simulink model "signal_processing"  (R2026a)
settings: Solver=ode4  StopTime=2.0  FixedStep=0.001
undefined symbols (not defined in the file): LPF_den, LPF_num, Sensor_Noise_Std, Ts
settings Model: Creator=anh  LastModifiedBy=anh
settings DataIOCC: ExternalInput=v_wheel_true_input, v_veh_zero  LoadExternalInput=on

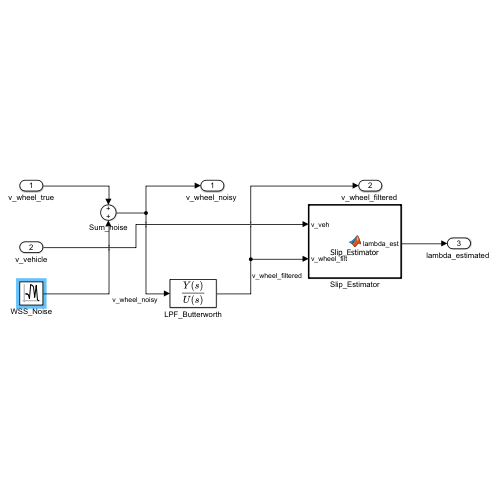
[thumbnail: Simulink's stored preview of the top-level diagram]
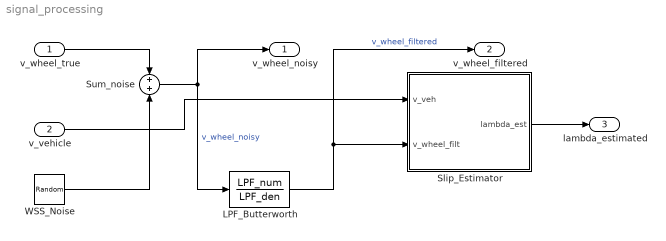
== system signal_processing ==
  v_wheel_true : Inport
  v_vehicle : Inport  Port=2
  LPF_Butterworth : TransferFcn  Numerator=LPF_num  Denominator=LPF_den
  Slip_Estimator : MATLAB Function  TreatAsAtomicUnit=on
  Sum_noise : Sum
  WSS_Noise : RandomNumber  Variance=Sensor_Noise_Std^2  SampleTime=Ts
  "v_wheel_noisy " : Outport
  "v_wheel_filtered " : Outport  Port=2
  "lambda_estimated " : Outport  Port=3
  wires:
  v_wheel_true/1 -> Sum_noise/1
  WSS_Noise/1 -> Sum_noise/2
  Sum_noise/1 -> LPF_Butterworth/1, "v_wheel_noisy "/1  "v_wheel_noisy"
  v_vehicle/1 -> Slip_Estimator/1(v_veh)
  LPF_Butterworth/1 -> "v_wheel_filtered "/1, Slip_Estimator/2(v_wheel_filt)  "v_wheel_filtered"
  Slip_Estimator/1(lambda_est) -> "lambda_estimated "/1

== matlab function signal_processing/Slip_Estimator ==
  data: v_veh input; lambda_est output; v_wheel_filt input
function lambda_est = Slip_Estimator(v_veh, v_wheel_filt)
% SLIP_ESTIMATOR Ước lượng slip ratio từ tín hiệu đã lọc nhiễu
% Có bảo vệ chống chia cho 0 khi xe dừng hẳn

if v_veh < 0.1
    lambda_est = 0.0;
else
    lambda_est = (v_veh - v_wheel_filt) / v_veh;
end

% Clamp về khoảng vật lý [0, 1]
lambda_est = max(0.0, min(1.0, lambda_est));
end
